simulink model "PMSM_SimModel_r2017b"  (R2017b)
settings: Solver=VariableStepAuto  StartTime=0.0  StopTime=4.0  MaxStep=1e-4  RelTol=1e-3
libraries: simulink x8, powerlib x7
settings Model: Creator=fei  LastModifiedBy=fei
settings SolverCC: ZeroCrossAlgorithm=Adaptive
settings DebuggingCC: IgnoredZcDiagnostic=none
settings SFSimCC: SimUseLocalCustomCode=on
settings RTWCC: RTWUseLocalCustomCode=on

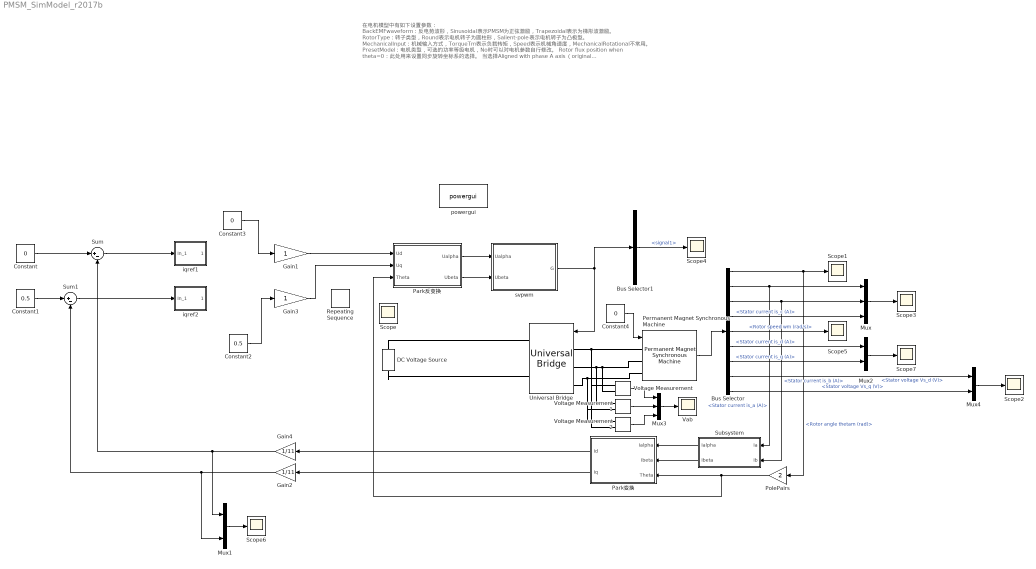
== system PMSM_SimModel_r2017b ==
  note: 在电机模型中有如下设置参数：
      | BackEMFwaveform：反电势波形，Sinusoidal表示PMSM为正弦激励，Trapezoidal表示为梯形波激励。
      | RotorType：转子类型，Round表示电机转子为圆柱形，Salient-pole表示电机转子为凸极型。
      | MechanicalInput：机械输入方式，TorqueTm表示负载转矩，Speed表示机械角速度，MechanicalRotational不常用。
      | PresetModel：电机类型，可选的功率等级电机，No时可以对电机参数自行修改。
      | Rotor flux position when theta=0：此处用来设置同步旋转坐标系的选择。
      | 当选择Aligned with phase A axis（original Park）时，表示同步旋转坐标系采用的是前面所讲的书本上常用坐标系（见图1-2）；
      | 当选择90degrees behind phase A axis（modified Park）时，表示同步旋转坐标系采用的是MATLAB自身所采用的坐标系（见图1-6）。
  Bus Selector : BusSelector  OutputSignals=Rotor angle thetam (rad),Stator current is_a (A),Stator current is_b (A),Stator current is_c (A),Rotor speed wm (rad/s),Stator current is_d (A),Stator current is_q (A),Stator voltage Vs_d (V),Stator voltage Vs_q (V)
  Bus Selector1 : BusSelector  OutputSignals=signal1
  Constant : Constant  Value=0
  Constant1 : Constant  Value=0.5
  Constant2 : Constant  Value=0.5
  Constant3 : Constant  Value=0
  Constant4 : Constant  Value=0
  DC Voltage Source : powerlib/Electrical Sources/DC Voltage Source  Amplitude=48  Measurements=None
  Gain1 : Gain
  Gain2 : Gain  Gain=1/11
  Gain3 : Gain
  Gain4 : Gain  Gain=1/11
  Mux : Mux  Inputs=3
  Mux1 : Mux  Inputs=2
  Mux2 : Mux  Inputs=2
  Mux3 : Mux  Inputs=3
  Mux4 : Mux  Inputs=2
  Park反变换 : Subsystem
  Park变换 : Subsystem
  Permanent Magnet Synchronous Machine : powerlib/Machines/Permanent Magnet Synchronous Machine  NbPhases=3  FluxDistribution=Sinusoidal  RotorType=Round  MechanicalLoad=Torque Tm  PresetModel=No  ShowDetailedParameters=on  MeasurementBus=off  Resistance=0.292  Inductance=8.5e-3  dqInductances=[8.5e-3,8.5e-3]  La=0.000240  MachineConstant=Flux linkage established by magnets (V.s)  Flux=0.1848  VoltageCst=31.4744  TorqueCst=0.26029  Flat=120  Mechanical=[0.00048 4.047e-05 0.939 0]  PolePairs=2  InitialConditions=[0,0, 0,0]  InitialConditions5ph=[0 0 0 0 0 0]  TsPowergui=0  TsBlock=-1  RefAngle=Aligned with phase A axis (original Park)
      settings: SourceProductName=Simscape Power Systems
  "PolePairs " : Gain  Gain=2
  Repeating Sequence : simulink/Sources/Repeating Sequence  rep_seq_t=[0 0.05]  rep_seq_y=[0 2*pi]
  Scope{,1..7} (8 alike) : Scope
  Subsystem : Subsystem
  Sum : Sum  Inputs=|+-
  Sum1 : Sum  Inputs=|+-
  Universal Bridge : powerlib/Power Electronics/Universal Bridge  Arms=3  SnubberResistance=1e5  SnubberCapacitance=inf  Device=MOSFET / Diodes  Ron=1e-3  Lon=0  ForwardVoltages="[  0  0  ]"  ForwardVoltage=0  GTOparameters=[ 10e-6 , 20e-6 ]  IGBTparameters=[ 1e-6 , 2e-6 ]  Measurements=None  Measurements_2=None  converterType=Rectifier
  Vab : Scope
  Voltage Measurement : powerlib/Measurements/Voltage Measurement  PhasorSimulation=off  OutputType=Complex  PSBequivalent=0
      settings: SourceProductName=Simscape Electrical
  Voltage Measurement1 : powerlib/Measurements/Voltage Measurement  PhasorSimulation=off  OutputType=Complex  PSBequivalent=0
      settings: SourceProductName=Simscape Electrical
  Voltage Measurement2 : powerlib/Measurements/Voltage Measurement  PhasorSimulation=off  OutputType=Complex  PSBequivalent=0
      settings: SourceProductName=Simscape Electrical
  iqref1 : Subsystem  mask(PI Controller){I=1, P=0.001, sat=[-500, 500]}
      mask prompts: I "Integral"; P "Proportional:"; sat "Minimum and maximum outputs:"
      mask init:
      | min=sat(1);max=sat(2);
      mask Display: disp('PI')
  iqref2 : Subsystem  mask(PI Controller){I=1, P=0.001, sat=[-500, 500]}
      mask prompts: I "Integral"; P "Proportional:"; sat "Minimum and maximum outputs:"
      mask init:
      | min=sat(1);max=sat(2);
      mask Display: disp('PI')
  powergui : powerlib/powergui  Priority=1  SimulationMode=Continuous  SampleTime=50e-6  frequency=10000  Iterations=50  frequencyindice=0  Pbase=100e6  ErrMax=1e-4  UnitsV=kV  UnitsW=MW  buscounter=0  FunctionMessages=off  echomessages=off  EnableUseOfTLC=off  CurrentSourceSwitches=off  DisableSnubberDevices=off  DisableRonSwitches=off  DisableVfSwitches=off  DisplayEquations=off  SolverType=Tustin/Backward Euler (TBE)  Interpol=off  ExternalGateDelay=off  methode=off  Ts=100  x0status=blocks  SPID=on  SwTol=0  HookPort=off  RestoreLinks=warning  ResistiveCurrentMeasurement=off  Frange=[0:2:500]  Ylog=off  Xlog=on  ShowGrid=off  save=off  variable=ZData  structure=0  ZoomFFT=off  StartTime=0.0  cycles=1  DisplayStyle=1  fundamental=60  FreqAxis=off  MaxFrequency=1000  frequencyindicesteady=1  RmsSteady=1  display=off
  svpwm : Subsystem
  wires:
  Park反变换/1(Ualpha) -> svpwm/1(Ualpha)
  Park反变换/2(Ubeta) -> svpwm/2(Ubeta)
  Permanent Magnet Synchronous Machine/1 -> Bus Selector/1
  Bus Selector/1 -> "PolePairs "/1, Scope1/1  "<Rotor angle thetam (rad)>"
  Bus Selector/2 -> Subsystem/1(Ia), Mux/1  "<Stator current is_a (A)>"
  Bus Selector/3 -> Subsystem/2(Ib), Mux/2  "<Stator current is_b (A)>"
  Bus Selector/4 -> Mux/3  "<Stator current is_c (A)>"
  Mux/1 -> Scope3/1
  svpwm/1(G) -> Bus Selector1/1, Universal Bridge/1
  Bus Selector1/1 -> Scope4/1  "<signal1>"
  Bus Selector/5 -> Scope5/1  "<Rotor speed wm (rad/s)>"
  Subsystem/1(Ialpha) -> Park变换/1(Ialpha)
  Subsystem/2("Ibeta ") -> Park变换/2(Ibeta)
  Mux1/1 -> Scope6/1
  Bus Selector/7 -> Mux2/2  "<Stator current is_q (A)>"
  Bus Selector/6 -> Mux2/1  "<Stator current is_d (A)>"
  Mux2/1 -> Scope7/1
  "PolePairs "/1 -> Park反变换/3(Theta), Park变换/3(Theta)
  Park变换/1(Id) -> Gain4/1
  Park变换/2(Iq) -> Gain2/1
  Gain3/1 -> Park反变换/2(Uq)
  Constant/1 -> Sum/1
  Constant1/1 -> Sum1/1
  Gain1/1 -> Park反变换/1(Ud)
  Sum/1 -> iqref1/1(In_1)
  Sum1/1 -> iqref2/1(In_1)
  Mux3/1 -> Vab/1
  Voltage Measurement/1 -> Mux3/1
  Voltage Measurement1/1 -> Mux3/2
  Voltage Measurement2/1 -> Mux3/3
  Bus Selector/8 -> Mux4/1  "<Stator voltage Vs_d (V)>"
  Mux4/1 -> Scope2/1
  Bus Selector/9 -> Mux4/2  "<Stator voltage Vs_q (V)>"
  Constant4/1 -> Permanent Magnet Synchronous Machine/1
  Gain2/1 -> Mux1/2, Sum1/2
  Gain4/1 -> Mux1/1, Sum/2
  Constant3/1 -> Gain1/1
  Constant2/1 -> Gain3/1
  connections:
  Universal Bridge/LConn1 -- Voltage Measurement2/LConn2 -- Voltage Measurement/LConn1 -- Permanent Magnet Synchronous Machine/LConn1
  Universal Bridge/LConn2 -- Voltage Measurement1/LConn1 -- Voltage Measurement/LConn2 -- Permanent Magnet Synchronous Machine/LConn2
  Universal Bridge/LConn3 -- Voltage Measurement1/LConn2 -- Voltage Measurement2/LConn1 -- Permanent Magnet Synchronous Machine/LConn3
  DC Voltage Source/LConn1 -- Universal Bridge/RConn2
  DC Voltage Source/RConn1 -- Universal Bridge/RConn1

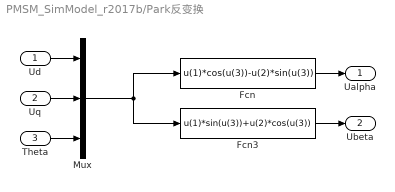
== system PMSM_SimModel_r2017b/Park反变换 ==
  Ud : Inport
  Uq : Inport  Port=2
  Theta : Inport  Port=3
  Fcn : Fcn  Expr=u(1)*cos(u(3))-u(2)*sin(u(3))
  Fcn3 : Fcn  Expr=u(1)*sin(u(3))+u(2)*cos(u(3))
  Mux : Mux  Inputs=3
  Ualpha : Outport
  Ubeta : Outport  Port=2
  wires:
  Ud/1 -> Mux/1
  Uq/1 -> Mux/2
  Theta/1 -> Mux/3
  Mux/1 -> Fcn3/1, Fcn/1
  Fcn3/1 -> Ubeta/1
  Fcn/1 -> Ualpha/1

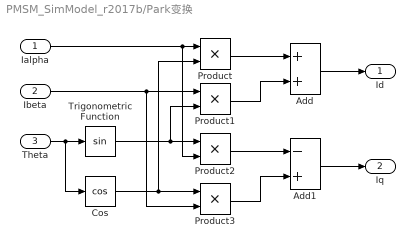
== system PMSM_SimModel_r2017b/Park变换 ==
  Ialpha : Inport
  Ibeta : Inport  Port=2
  Theta : Inport  Port=3
  Add : Sum
  Add1 : Sum  Inputs=-+
  Cos : Trigonometry  Operator=cos
  Product{,1..3} (4 alike) : Product
  Trigonometric Function : Trigonometry
  Id : Outport
  Iq : Outport  Port=2
  wires:
  Ialpha/1 -> Product2/2, Product/1
  Ibeta/1 -> Product3/2, Product1/1
  Theta/1 -> Cos/1, Trigonometric Function/1
  Trigonometric Function/1 -> Product1/2, Product2/1
  Cos/1 -> Product/2, Product3/1
  Add1/1 -> Iq/1
  Add/1 -> Id/1
  Product/1 -> Add/1
  Product1/1 -> Add/2
  Product2/1 -> Add1/1
  Product3/1 -> Add1/2

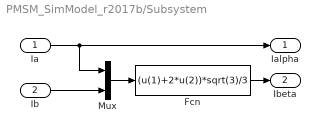
== system PMSM_SimModel_r2017b/Subsystem ==
  Ia : Inport
  Ib : Inport  Port=2
  Fcn : Fcn  Expr=(u(1)+2*u(2))*sqrt(3)/3
  Mux : Mux  Inputs=2
  Ialpha : Outport
  "Ibeta " : Outport  Port=2
  wires:
  Ia/1 -> Mux/1, Ialpha/1
  Ib/1 -> Mux/2
  Mux/1 -> Fcn/1
  Fcn/1 -> "Ibeta "/1

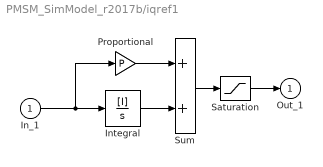
== system PMSM_SimModel_r2017b/iqref1 ==
  In_1 : Inport
  Integral : TransferFcn  Numerator=[I]  Denominator=[1 0]
  Proportional : Gain  Gain=P  SaturateOnIntegerOverflow=on  OutDataTypeStr=Inherit: Same as input  ParamDataTypeStr=Inherit: Same as input
  Saturation : Saturate  UpperLimit=max  LowerLimit=min
  Sum : Sum  SaturateOnIntegerOverflow=on  InputSameDT=on  OutDataTypeStr=Inherit: Same as first input
  Out_1 : Outport  InitialOutput=0
  wires:
  Saturation/1 -> Out_1/1
  Sum/1 -> Saturation/1
  Proportional/1 -> Sum/1
  In_1/1 -> Proportional/1, Integral/1
  Integral/1 -> Sum/2

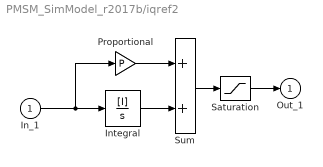
== system PMSM_SimModel_r2017b/iqref2 ==
  In_1 : Inport
  Integral : TransferFcn  Numerator=[I]  Denominator=[1 0]
  Proportional : Gain  Gain=P  SaturateOnIntegerOverflow=on  OutDataTypeStr=Inherit: Same as input  ParamDataTypeStr=Inherit: Same as input
  Saturation : Saturate  UpperLimit=max  LowerLimit=min
  Sum : Sum  SaturateOnIntegerOverflow=on  InputSameDT=on  OutDataTypeStr=Inherit: Same as first input
  Out_1 : Outport  InitialOutput=0
  wires:
  Saturation/1 -> Out_1/1
  Sum/1 -> Saturation/1
  Proportional/1 -> Sum/1
  In_1/1 -> Proportional/1, Integral/1
  Integral/1 -> Sum/2

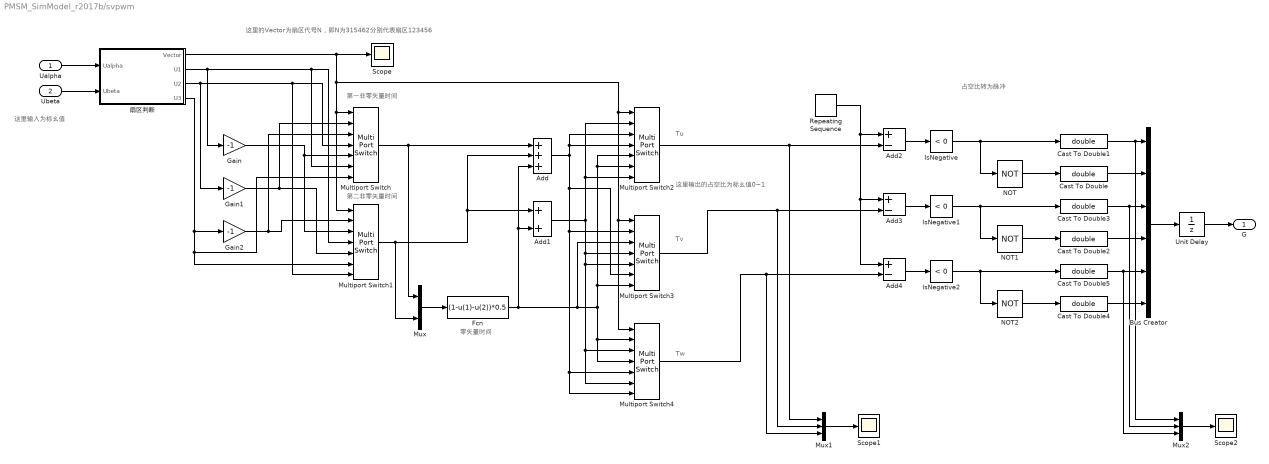
== system PMSM_SimModel_r2017b/svpwm ==
  note: Tu
  note: 这里输出的占空比为标幺值0~1
  note: 这里输入为标幺值
  note: 零矢量时间
  note: 第二非零矢量时间
  note: 第一非零矢量时间
  note: 这里的Vector为扇区代号N，即N为315462分别代表扇区123456
  note: Tv
  note: Tw
  note: 占空比转为脉冲
  Ualpha : Inport
  Ubeta : Inport  Port=2
  Add : Sum  Inputs=+++
  Add1 : Sum
  Add2 : Sum  Inputs=+-
  Add3 : Sum  Inputs=+-
  Add4 : Sum  Inputs=+-
  Bus Creator : BusCreator  Inputs=6
  Cast To Double{,1..5} (6 alike) : DataTypeConversion  OutDataTypeStr=double
  Fcn : Fcn  Expr=(1-u(1)-u(2))*0.5
  Gain : Gain  Gain=-1
  Gain1 : Gain  Gain=-1
  Gain2 : Gain  Gain=-1
  IsNegative : simulink/Logic and Bit Operations/Compare To Zero  relop=<  OutDataTypeStr=boolean
  IsNegative1 : simulink/Logic and Bit Operations/Compare To Zero  relop=<  OutDataTypeStr=boolean
  IsNegative2 : simulink/Logic and Bit Operations/Compare To Zero  relop=<  OutDataTypeStr=boolean
  Multiport Switch{,1..4} (5 alike) : MultiPortSwitch  Inputs=6
  Mux : Mux  Inputs=2
  Mux1 : Mux  Inputs=3
  Mux2 : Mux  Inputs=3
  NOT : Logic  Operator=NOT  IconShape=distinctive  AllPortsSameDT=off  OutDataTypeStr=boolean
  NOT1 : Logic  Operator=NOT  IconShape=distinctive  AllPortsSameDT=off  OutDataTypeStr=boolean
  NOT2 : Logic  Operator=NOT  IconShape=distinctive  AllPortsSameDT=off  OutDataTypeStr=boolean
  Repeating Sequence : simulink/Sources/Repeating Sequence  rep_seq_t=[0 0.0005 0.001]  rep_seq_y=[0 1 0]
  Scope : Scope
  Scope1 : Scope
  Scope2 : Scope
  Unit Delay : UnitDelay  SampleTime=-1
  扇区判断 : Subsystem
  G : Outport
  wires:
  Ubeta/1 -> 扇区判断/2(Ubeta)
  Ualpha/1 -> 扇区判断/1(Ualpha)
  扇区判断/1(Vector) -> Multiport Switch3/1, Multiport Switch4/1, Multiport Switch2/1, Multiport Switch1/1, Multiport Switch/1, Scope/1
  扇区判断/2(U1) -> Multiport Switch1/4, Multiport Switch/6, Gain/1
  扇区判断/3(U2) -> Multiport Switch/4, Multiport Switch1/7, Gain1/1
  扇区判断/4(U3) -> Multiport Switch/7, Multiport Switch1/6, Gain2/1
  Gain1/1 -> Multiport Switch1/5, Multiport Switch/2
  Gain2/1 -> Multiport Switch/3, Multiport Switch1/2
  Gain/1 -> Multiport Switch/5, Multiport Switch1/3
  Multiport Switch/1 -> Add/1, Mux/1
  Multiport Switch1/1 -> Add1/1, Add/2, Mux/2
  Mux/1 -> Fcn/1
  Fcn/1 -> Add1/2, Add/3, Multiport Switch4/4, Multiport Switch4/2, Multiport Switch3/7, Multiport Switch2/6, Multiport Switch2/5, Multiport Switch3/3
  Add1/1 -> Multiport Switch4/6, Multiport Switch4/3, Multiport Switch3/5, Multiport Switch3/4, Multiport Switch2/7, Multiport Switch2/2
  Add/1 -> Multiport Switch2/4, Multiport Switch2/3, Multiport Switch3/6, Multiport Switch4/7, Multiport Switch4/5, Multiport Switch3/2
  Multiport Switch4/1 -> Mux1/3, Add4/2
  Unit Delay/1 -> G/1
  Cast To Double1/1 -> Mux2/1, Bus Creator/1
  IsNegative1/1 -> NOT1/1, Cast To Double3/1
  Cast To Double2/1 -> Bus Creator/4
  Cast To Double3/1 -> Mux2/2, Bus Creator/3
  Add4/1 -> IsNegative2/1
  Cast To Double4/1 -> Bus Creator/6
  Cast To Double5/1 -> Mux2/3, Bus Creator/5
  IsNegative/1 -> NOT/1, Cast To Double1/1
  Add3/1 -> IsNegative1/1
  Bus Creator/1 -> Unit Delay/1
  IsNegative2/1 -> NOT2/1, Cast To Double5/1
  Repeating Sequence/1 -> Add4/1, Add3/1, Add2/1
  Cast To Double/1 -> Bus Creator/2
  NOT2/1 -> Cast To Double4/1
  Add2/1 -> IsNegative/1
  NOT/1 -> Cast To Double/1
  NOT1/1 -> Cast To Double2/1
  Multiport Switch2/1 -> Mux1/1, Add2/2
  Multiport Switch3/1 -> Mux1/2, Add3/2
  Mux1/1 -> Scope1/1
  Mux2/1 -> Scope2/1

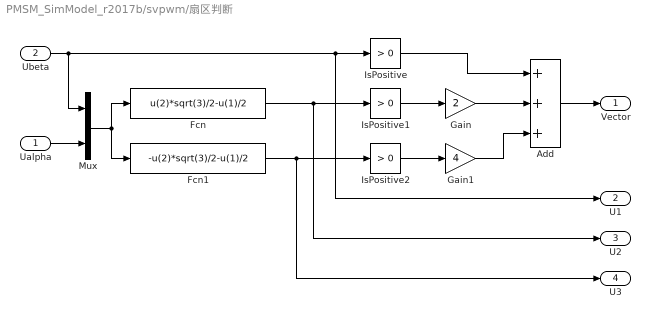
== system PMSM_SimModel_r2017b/svpwm/扇区判断 ==
  Ualpha : Inport
  Ubeta : Inport  Port=2
  Add : Sum  Inputs=+++
  Fcn : Fcn  Expr=u(2)*sqrt(3)/2-u(1)/2
  Fcn1 : Fcn  Expr=-u(2)*sqrt(3)/2-u(1)/2
  Gain : Gain  Gain=2
  Gain1 : Gain  Gain=4
  IsPositive : simulink/Logic and Bit Operations/Compare To Zero  relop=>  OutDataTypeStr=boolean
  IsPositive1 : simulink/Logic and Bit Operations/Compare To Zero  relop=>  OutDataTypeStr=boolean
  IsPositive2 : simulink/Logic and Bit Operations/Compare To Zero  relop=>  OutDataTypeStr=boolean
  Mux : Mux  Inputs=2
  Vector : Outport
  U1 : Outport  Port=2
  U2 : Outport  Port=3
  U3 : Outport  Port=4
  wires:
  Mux/1 -> Fcn1/1, Fcn/1
  Ualpha/1 -> Mux/2
  IsPositive2/1 -> Gain1/1
  Fcn/1 -> U2/1, IsPositive1/1
  Fcn1/1 -> U3/1, IsPositive2/1
  Gain1/1 -> Add/3
  IsPositive1/1 -> Gain/1
  Gain/1 -> Add/2
  IsPositive/1 -> Add/1
  Add/1 -> Vector/1
  Ubeta/1 -> U1/1, IsPositive/1, Mux/1
